simulink model "frame_sync_detector"  (R2020b)
settings: Solver=VariableStepAuto  StartTime=0.0  StopTime=10  FixedStep=0.01  RelTol=1e-3
values from neighbouring files (symbols this model uses):
  pPLHeader = pPLHeader.'    [data.m]
libraries: dspsrcs4 x1, dsphdlmathfun x1
settings Model: SimulationMode=accelerator  Creator=23947  LastModifiedBy=23947
settings GRTTargetCC: RTWCAPISignals=on  RTWCAPIParams=on

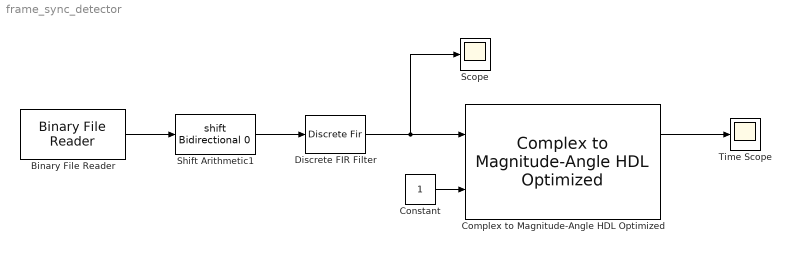
== system frame_sync_detector ==
  Binary File Reader : dspsrcs4/Binary File Reader  Filename=C:\Users\23947\Desktop\now\Assignment\DSP\frame_sync_detector\data.bin  HeaderStructure=struct([])  DataType=int16  SamplesPerFrame=1  IsDataComplex=on  NumChannels=1  OutputEOF=off  SampleTime=1/90e3  SimulateUsing=Code generation
      settings: SourceProductBaseCode=DS
  Complex to Magnitude-Angle HDL Optimized : dsphdlmathfun/Complex to Magnitude-Angle HDL Optimized  NumIterationsSource=Auto  NumIterations=10  OutputFormat=Magnitude  AngleFormat=Normalized  ScaleOutput=on  SimulateUsing=Code generation
      settings: SourceProductBaseCode=DS
  Constant : Constant  VectorParams1D=off  OutDataTypeStr=boolean
  Discrete FIR Filter : DiscreteFir  Coefficients=flip(conj(pPLHeader)) .* sqrt(2)  CoefDataTypeStr=fixdt(1,2,0)
  Scope : Scope
  Shift Arithmetic1 : ArithShift  BinPtShiftNumber=-14
  Time Scope : Scope
  wires:
  Constant/1 -> Complex to Magnitude-Angle HDL Optimized/2
  Binary File Reader/1 -> Shift Arithmetic1/1
  Shift Arithmetic1/1 -> Discrete FIR Filter/1
  Complex to Magnitude-Angle HDL Optimized/1 -> Time Scope/1
  Discrete FIR Filter/1 -> Scope/1, Complex to Magnitude-Angle HDL Optimized/1
